simulink model "Active_Body_Control_stud"  (R2016b)
settings: Solver=ode45  StartTime=0.0  StopTime=50  FixedStep=0.01  RelTol=1e-3  EnableMultiTasking=on
values from neighbouring files (symbols this model uses):
  A_cyl = pi*(D_kolben^2)/4    (= 0.000314159265359)    [Active_Body_Control_param_stud.m]
  alpha_K_blende = 0.6    [Active_Body_Control_param_stud.m]
  bore_max = 20e-6    (= 2e-05)    [Active_Body_Control_param_stud.m]
  c = 400    [Active_Body_Control_param_stud.m]
  c_A = 19000    [Active_Body_Control_param_stud.m]
  c_R = 190500    [Active_Body_Control_param_stud.m]
  d_A = 1100    [Active_Body_Control_param_stud.m]
  delta_y_s = 0.005    [Active_Body_Control_param_stud.m]
  g = 9.81    [Active_Body_Control_param_stud.m]
  Km = 1    [Active_Body_Control_param_stud.m]
  L = 1e-5    (= 1e-05)    [Active_Body_Control_param_stud.m]
  m_A = 200    [Active_Body_Control_param_stud.m]
  m_R = 40    [Active_Body_Control_param_stud.m]
  m_va = 0.1    [Active_Body_Control_param_stud.m]
  P_pump = 150e5    (= 15000000)    [Active_Body_Control_param_stud.m]
  R = 1.2    [Active_Body_Control_param_stud.m]
  rho = 880    [Active_Body_Control_param_stud.m]
  s_max_va = 0.020    (= 0.02)    [Active_Body_Control_param_stud.m]
settings Model: Creator=da.klinder  LastModifiedBy=ti.unbehaun
settings DataIOCC: LimitDataPoints=on  SaveFormat=Array  SignalLoggingSaveFormat=ModelDataLogs
settings OptimizationCC: ExpressionDepthLimit=2147483647  LifeSpan=inf
settings DebuggingCC: UnderspecifiedInitializationDetection=Classic  MergeDetectMultiDrivingBlocksExec=none  SolverPrmCheckMsg=warning  FcnCallInpInsideContextMsg=warning  StateNameClashWarn=warning  SFUnexpectedBacktrackingDiag=warning  SFNoUnconditionalDefaultTransitionDiag=warning  SFExecutionAtInitializationDiag=none
settings HardwareCC: ProdBitPerPointer=32  ProdBitPerSizeT=32  ProdBitPerPtrDiffT=32  ProdLargestAtomicFloat=None  ProdIntDivRoundTo=Undefined  ProdEndianess=Unspecified  ProdWordSize=32  ProdHWDeviceType=32-bit Generic
settings ModelReferenceCC: PropagateSignalLabelsOutOfModel=off
settings GRTTargetCC: TargetLangStandard=C89/C90 (ANSI)  GeneratePreprocessorConditionals=Disable all  CombineOutputUpdateFcns=off  GRTInterface=on
settings ConfigComp: CovMetricSettings=dw  CovHtmlReporting=on  CovSaveCumulativeToWorkspaceVar=on  CovSaveSingleToWorkspaceVar=on  CovExternalEMLEnable=off

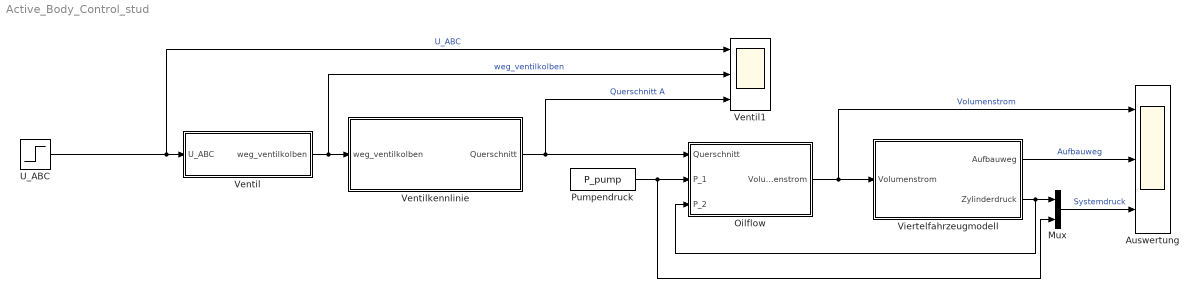
== system Active_Body_Control_stud ==
  Auswertung : Scope  NumInputPorts=3
  Mux : Mux  Inputs=2
  Oilflow : Subsystem
  Pumpendruck : Constant  Value=P_pump
  U_ABC : Step  Time=5  After=5  SampleTime=0
  Ventil : Subsystem
  Ventil1 : Scope  NumInputPorts=3
  Ventilkennlinie : Subsystem
  Viertelfahrzeugmodell : Subsystem
  wires:
  Ventil/1(weg_ventilkolben) -> Ventilkennlinie/1(weg_ventilkolben), Ventil1/2  "weg_ventilkolben"
  Pumpendruck/1 -> Mux/2, Oilflow/2(P_1)
  Ventilkennlinie/1(Querschnitt) -> Ventil1/3, Oilflow/1(Querschnitt)  "Querschnitt A"
  Oilflow/1(Volumenstrom) -> Viertelfahrzeugmodell/1(Volumenstrom), Auswertung/1  "Volumenstrom"
  Viertelfahrzeugmodell/2(Zylinderdruck) -> Mux/1, Oilflow/3(P_2)
  Mux/1 -> Auswertung/3  "Systemdruck"
  U_ABC/1 -> Ventil1/1, Ventil/1(U_ABC)  "U_ABC"
  Viertelfahrzeugmodell/1(Aufbauweg) -> Auswertung/2  "Aufbauweg"

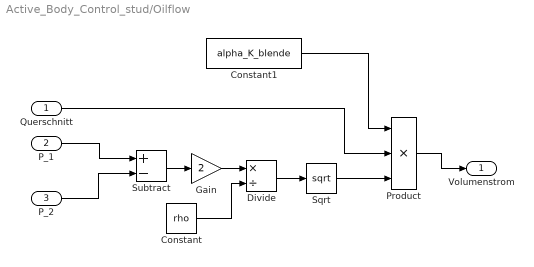
== system Active_Body_Control_stud/Oilflow ==
  Querschnitt : Inport
  P_1 : Inport  Port=2
  P_2 : Inport  Port=3
  Constant : Constant  Value=rho
  Constant1 : Constant  Value=alpha_K_blende
  Divide : Product  Inputs=*/
  Gain : Gain  Gain=2
  Product : Product  Inputs=3
  Sqrt : Sqrt  SaturateOnIntegerOverflow=on
  Subtract : Sum  Inputs=+-
  Volumenstrom : Outport
  wires:
  P_1/1 -> Subtract/1
  P_2/1 -> Subtract/2
  Subtract/1 -> Gain/1
  Gain/1 -> Divide/1
  Constant/1 -> Divide/2
  Divide/1 -> Sqrt/1
  Sqrt/1 -> Product/3
  Querschnitt/1 -> Product/2
  Constant1/1 -> Product/1
  Product/1 -> Volumenstrom/1

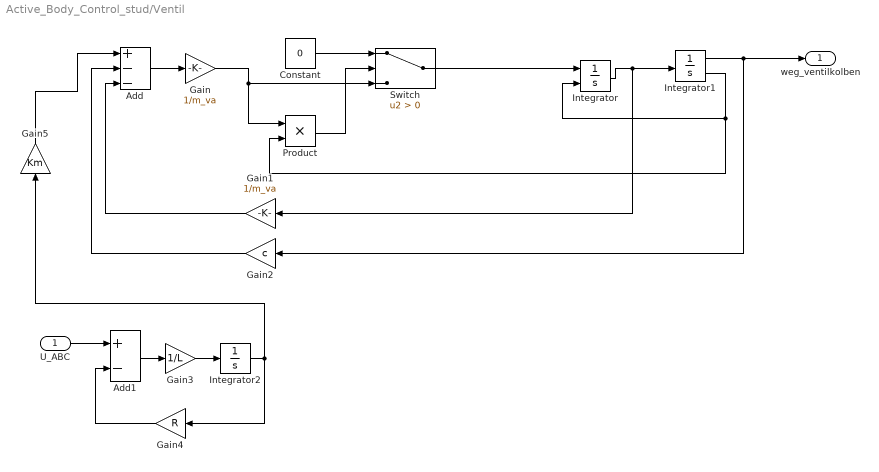
== system Active_Body_Control_stud/Ventil ==
  U_ABC : Inport
  Add : Sum  Inputs=+--
  Add1 : Sum  Inputs=+-
  Constant : Constant  Value=0
  Gain : Gain  Gain=1/m_va
  Gain1 : Gain  Gain=1/m_va
  Gain2 : Gain  Gain=c
  Gain3 : Gain  Gain=1/L
  Gain4 : Gain  Gain=R
  Gain5 : Gain  Gain=Km
  Integrator : Integrator  ExternalReset=either
  Integrator1 : Integrator  LimitOutput=on  UpperSaturationLimit=s_max_va  LowerSaturationLimit=-s_max_va  ShowSaturationPort=on
  Integrator2 : Integrator
  Product : Product
  Switch : Switch  Criteria=u2 > Threshold
  weg_ventilkolben : Outport
  wires:
  Add/1 -> Gain/1
  Gain/1 -> Product/1, Switch/3
  Integrator/1 -> Gain1/1, Integrator1/1
  Gain1/1 -> Add/3
  Integrator1/1 -> Gain2/1, weg_ventilkolben/1
  Gain2/1 -> Add/2
  Integrator2/1 -> Gain4/1, Gain5/1
  U_ABC/1 -> Add1/1
  Add1/1 -> Gain3/1
  Gain3/1 -> Integrator2/1
  Gain4/1 -> Add1/2
  Gain5/1 -> Add/1
  Integrator1/2 -> Product/2, Integrator/2
  Switch/1 -> Integrator/1
  Product/1 -> Switch/2
  Constant/1 -> Switch/1

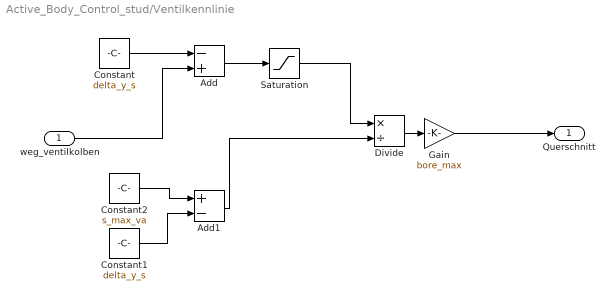
== system Active_Body_Control_stud/Ventilkennlinie ==
  weg_ventilkolben : Inport
  Add : Sum  Inputs=-+
  Add1 : Sum  Inputs=+-
  Constant : Constant  Value=delta_y_s
  Constant1 : Constant  Value=delta_y_s
  Constant2 : Constant  Value=s_max_va
  Divide : Product  Inputs=*/
  Gain : Gain  Gain=bore_max
  Saturation : Saturate  UpperLimit=inf  LowerLimit=0
  Querschnitt : Outport
  wires:
  weg_ventilkolben/1 -> Add/2
  Constant/1 -> Add/1
  Add/1 -> Saturation/1
  Add1/1 -> Divide/2
  Constant1/1 -> Add1/2
  Constant2/1 -> Add1/1
  Divide/1 -> Gain/1
  Gain/1 -> Querschnitt/1
  Saturation/1 -> Divide/1

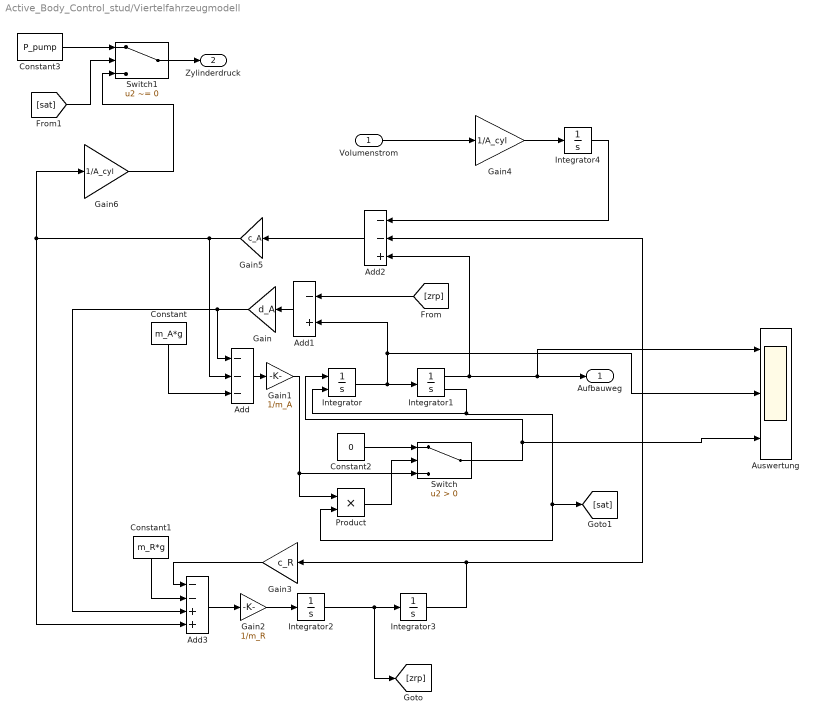
== system Active_Body_Control_stud/Viertelfahrzeugmodell ==
  Volumenstrom : Inport
  Add : Sum  Inputs=---
  Add1 : Sum  Inputs=-+
  Add2 : Sum  Inputs=--+
  Add3 : Sum  Inputs=--++
  Auswertung : Scope  NumInputPorts=3
  Constant : Constant  Value=m_A*g
  Constant1 : Constant  Value=m_R*g
  Constant2 : Constant  Value=0
  Constant3 : Constant  Value=P_pump
  Gain : Gain  Gain=d_A
  Gain1 : Gain  Gain=1/m_A
  Gain2 : Gain  Gain=1/m_R
  Gain3 : Gain  Gain=c_R
  Gain4 : Gain  Gain=1/A_cyl
  Gain5 : Gain  Gain=c_A
  Gain6 : Gain  Gain=1/A_cyl
  Integrator : Integrator  ExternalReset=either
  Integrator1 : Integrator  LimitOutput=on  UpperSaturationLimit=0.3  LowerSaturationLimit=0  ShowSaturationPort=on
  Integrator2 : Integrator
  Integrator3 : Integrator
  Integrator4 : Integrator
  Product : Product
  Switch : Switch  Criteria=u2 > Threshold
  Switch1 : Switch  Criteria=u2 ~= 0
  Aufbauweg : Outport
  Zylinderdruck : Outport  Port=2
  wires:
  Integrator/1 -> Auswertung/2, Add1/2, Integrator1/1
  Add1/1 -> Gain/1
  Integrator2/1 -> [zrp], Integrator3/1
  Gain/1 -> Add3/3, Add/1
  Add2/1 -> Gain5/1
  Constant/1 -> Add/3
  Integrator3/1 -> Add2/2, Gain3/1
  Add/1 -> Gain1/1
  Gain2/1 -> Integrator2/1
  Add3/1 -> Gain2/1
  Gain3/1 -> Add3/1
  Constant1/1 -> Add3/2
  Gain5/1 -> Add3/4, Gain6/1, Add/2
  Gain6/1 -> Switch1/3
  Integrator1/1 -> Add2/3, Auswertung/1, Aufbauweg/1
  Gain1/1 -> Switch/3, Product/1
  Integrator1/2 -> [sat], Product/2, Integrator/2
  Switch/1 -> Auswertung/3, Integrator/1
  Product/1 -> Switch/2
  Constant2/1 -> Switch/1
  Gain4/1 -> Integrator4/1
  Volumenstrom/1 -> Gain4/1
  Integrator4/1 -> Add2/1
  [zrp] -> Add1/1
  Constant3/1 -> Switch1/1
  [sat] -> Switch1/2
  Switch1/1 -> Zylinderdruck/1
